simulink model "SMC_c_2015a"  (R2015a)
settings: Solver=ode45  SolverMode=SingleTasking  StartTime=0.0  StopTime=30  FixedStep=8e-5  RelTol=1e-3
settings Model: CovMetricSettings=dwe  CovHtmlReporting=off  covSaveCumulativeToWorkspaceVar=off  CovSaveSingleToWorkspaceVar=off  CovExternalEMLEnable=on  Creator=seumagal  LastModifiedBy=zoero
settings DataIOCC: LimitDataPoints=off  SaveFormat=Dataset
settings DebuggingCC: SFUnexpectedBacktrackingDiag=error  SFNoUnconditionalDefaultTransitionDiag=error
settings HardwareCC: ProdBitPerPointer=64  ProdLargestAtomicFloat=Float  ProdIntDivRoundTo=Zero  ProdEndianess=LittleEndian  ProdHWDeviceType=Specified
settings ModelReferenceCC: PropagateSignalLabelsOutOfModel=on
settings GRTTargetCC: TargetLangStandard=C99 (ISO)  GeneratePreprocessorConditionals=Use local settings

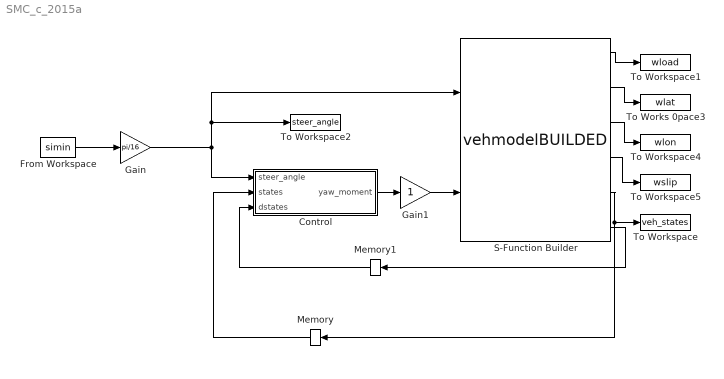
== system SMC_c_2015a ==
  "Control " : Subsystem  TreatAsAtomicUnit=on
  From Workspace : FromWorkspace  VariableName=simin  SampleTime=0
  Gain : Gain  Gain=pi/16
  Gain1 : Gain
  Memory : Memory  X0=[0,18,0,0,0]
  Memory1 : Memory
  S-Function Builder : S-Function  InitFcn=try, set_param(gcb,'FunctionName','vehmodelBUILDED'), end  FunctionName=vehmodelBUILDED  Parameters=params  SFunctionModules=vehmodelBUILDED_wrapper  mask(S-Function Builder){}
      mask help: Simulink:masks:SFunctionBuilder_MD
      mask init:
      | val = [[.9  0.75 0.75 1 1 .9 .9 1]',[1 1 0.75 0.75 .9 .9 1 .9]'];try , sys = get_param(gcb,'SfunBuilderFcnName');if isempty(sys), sys = get_param(gcb,'FunctionName'); end,catch, sys = get_param(gcb,'FunctionName'); end
      settings: CopyFcn=set_param(gcbh,'LinkStatus','none')  PreSaveFcn=try, set_param(gcb,'FunctionName','vehmodelBUILDED'), end  OpenFcn=sfunctionwizard(gcbh)
      mask Display:
      | plot(val(:,1),val(:,2))
      | disp(sys)
      | port_label('input',1,'inSteer')
      | port_label('input',2,'inMz')
      | port_label('output',1,'outFz')
      | port_label('output',2,'outFy')
      | port_label('output',3,'outFx')
      | port_label('output',4,'outSlip')
      | port_label('output',5,'outStates')
      | port_label('output',6,'outDStates')
  To Works 0pace3 : ToWorkspace  VariableName=wlat  SaveFormat=Timeseries  SampleTime=-1
  To Workspace : ToWorkspace  VariableName=veh_states  SaveFormat=Timeseries  SampleTime=-1
  To Workspace1 : ToWorkspace  VariableName=wload  SaveFormat=Timeseries  SampleTime=-1
  To Workspace2 : ToWorkspace  VariableName=steer_angle  SaveFormat=Timeseries  SampleTime=-1
  To Workspace4 : ToWorkspace  VariableName=wlon  SaveFormat=Timeseries  SampleTime=-1
  To Workspace5 : ToWorkspace  VariableName=wslip  SaveFormat=Timeseries  SampleTime=-1
  wires:
  From Workspace/1 -> Gain/1
  Gain/1 -> S-Function Builder/1, To Workspace2/1, "Control "/1(steer_angle)
  Memory/1 -> "Control "/2(states)
  S-Function Builder/5 -> Memory/1, To Workspace/1
  S-Function Builder/1 -> To Workspace1/1
  S-Function Builder/3 -> To Workspace4/1
  S-Function Builder/2 -> To Works 0pace3/1
  S-Function Builder/4 -> To Workspace5/1
  S-Function Builder/6 -> Memory1/1
  Memory1/1 -> "Control "/3(dstates)
  "Control "/1(yaw_moment) -> Gain1/1
  Gain1/1 -> S-Function Builder/2

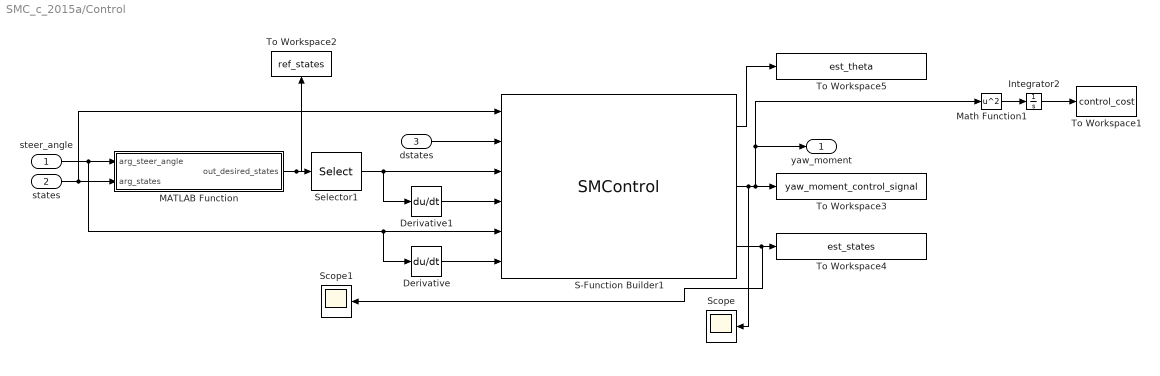
== system SMC_c_2015a/Control  ==
  steer_angle : Inport
  states : Inport  Port=2
  dstates : Inport  Port=3
  Derivative : Derivative
  Derivative1 : Derivative
  Integrator2 : Integrator
  MATLAB Function : MATLAB Function  TreatAsAtomicUnit=on
  Math Function1 : Math  Operator=square  SaturateOnIntegerOverflow=on
  S-Function Builder1 : S-Function  InitFcn=try, set_param(gcb,'FunctionName','SMControl'), end  FunctionName=SMControl  Parameters=paramssmc  SFunctionModules=SMControl_wrapper  mask(S-Function Builder){}
      mask help: Simulink:masks:SFunctionBuilder_MD
      mask init: same as SMC_c_2015a/S-Function Builder
      settings: CopyFcn=set_param(gcbh,'LinkStatus','none')  PreSaveFcn=try, set_param(gcb,'FunctionName','SMControl'), end  OpenFcn=sfunctionwizard(gcbh)
      mask Display:
      | plot(val(:,1),val(:,2))
      | disp(sys)
      | port_label('input',1,'inStates')
      | port_label('input',2,'inDStates')
      | port_label('input',3,'inDesiredYaw')
      | port_label('input',4,'inDDesiredYaw')
      | port_label('input',5,'inSteer')
      | port_label('input',6,'inDSteer')
      | port_label('output',1,'outTheta')
      | port_label('output',2,'outControl')
      | port_label('output',3,'outEstState')
  Scope : Scope
      settings: YMin=-15000  YMax=15000
  Scope1 : Scope
      settings: YMin=-1  YMax=17
  Selector1 : Selector  InputPortWidth=4  Indices=[2]
  To Workspace1 : ToWorkspace  VariableName=control_cost  SaveFormat=Timeseries  SampleTime=-1
      settings: MaxDataPoints=1
  To Workspace2 : ToWorkspace  VariableName=ref_states  SaveFormat=Timeseries  SampleTime=-1
      settings: MaxDataPoints=Inf
  To Workspace3 : ToWorkspace  VariableName=yaw_moment_control_signal  SaveFormat=Timeseries  SampleTime=-1
      settings: MaxDataPoints=Inf
  To Workspace4 : ToWorkspace  VariableName=est_states  SaveFormat=Timeseries  SampleTime=-1
      settings: MaxDataPoints=Inf
  To Workspace5 : ToWorkspace  VariableName=est_theta  SaveFormat=Timeseries  SampleTime=-1
      settings: MaxDataPoints=Inf
  yaw_moment : Outport
  wires:
  Math Function1/1 -> Integrator2/1
  Integrator2/1 -> To Workspace1/1
  states/1 -> S-Function Builder1/1, MATLAB Function/2(arg_states)
  MATLAB Function/1(out_desired_states) -> To Workspace2/1, Selector1/1
  Selector1/1 -> Derivative1/1, S-Function Builder1/3
  dstates/1 -> S-Function Builder1/2
  steer_angle/1 -> Derivative/1, S-Function Builder1/5, MATLAB Function/1(arg_steer_angle)
  S-Function Builder1/2 -> Scope/1, Math Function1/1, yaw_moment/1, To Workspace3/1
  S-Function Builder1/3 -> Scope1/1, To Workspace4/1
  S-Function Builder1/1 -> To Workspace5/1
  Derivative/1 -> S-Function Builder1/6
  Derivative1/1 -> S-Function Builder1/4

== matlab function SMC_c_2015a/Control /MATLAB Function ==
  data: arg_steer_angle input; out_desired_states output; arg_states input
    function  out_desired_states  = desired_states( arg_steer_angle, arg_states )

persistent mu_g;
persistent Ku;
persistent l;
if isempty(Ku)
    modelParams = coder.load( 'modelParam.mat' );
    Ku = modelParams.Ku;
    mu_g = modelParams.friction_coefficient*modelParams.g;
    l = modelParams.l;
end

long_speed = arg_states(2);
desired_yaw_rate =  long_speed*arg_steer_angle/(l + Ku*long_speed.^2);
max_yaw_rate = abs(mu_g/long_speed);

if abs(desired_yaw_rate) > max_yaw_rate
    desired_yaw_rate = max_yaw_rate*sign(desired_yaw_rate);
end
    
out_desired_states = [0; desired_yaw_rate; 0; 0 ];

end
